simulink model "assembly_line"  (R2024b)
settings: Solver=VariableStepAuto  StartTime=0.0  StopTime=10.0  RelTol=1e-3
libraries: testLib x5
settings Model: Creator=AK123700  LastModifiedBy=AK123700

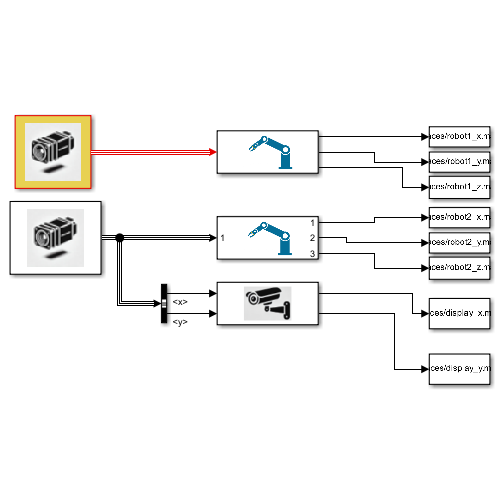
[thumbnail: Simulink's stored preview of the top-level diagram]
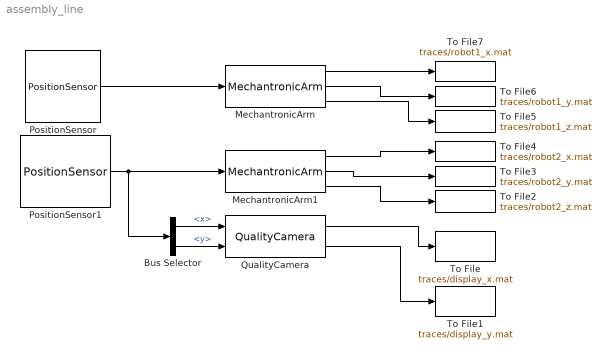
== system assembly_line ==
  Bus Selector : BusSelector  OutputSignals=x,y
  MechantronicArm : testLib/MechantronicArm  SystemSampleTime=-1  VariantActivationTime=update diagram  AllowFlexibleInterface=on  Latency=0  AutoFrameSizeCalculation=off
      mask Display: image('robot-icon.png', [0,0,0,0,80,80]);
  MechantronicArm1 : testLib/MechantronicArm  SystemSampleTime=-1  VariantActivationTime=update diagram  AllowFlexibleInterface=on  Latency=0  AutoFrameSizeCalculation=off
      mask Display: image('robot-icon.png', [0,0,0,0,80,80]);
  PositionSensor : testLib/PositionSensor  SystemSampleTime=-1  VariantActivationTime=update diagram  AllowFlexibleInterface=on  Latency=0  AutoFrameSizeCalculation=off
      mask Display: image('position-icon.png', [0,0,0,0,80,80]);
  PositionSensor1 : testLib/PositionSensor  SystemSampleTime=-1  VariantActivationTime=update diagram  AllowFlexibleInterface=on  Latency=0  AutoFrameSizeCalculation=off
      mask Display: image('position-icon.png', [0,0,0,0,80,80]);
  QualityCamera : testLib/QualityCamera  SystemSampleTime=-1  VariantActivationTime=update diagram  AllowFlexibleInterface=on  Latency=0  AutoFrameSizeCalculation=off
      mask Display: image('camera-icon.png', [0,0,0,0,80,80]);
  To File : ToFile  Filename=traces/display_x.mat  MatrixName=display_x_final  SaveFormat=Timeseries
  To File1 : ToFile  Filename=traces/display_y.mat  MatrixName=display_y_final  SaveFormat=Timeseries
  To File2 : ToFile  Filename=traces/robot2_z.mat  MatrixName=robot2_z_final  SaveFormat=Timeseries
  To File3 : ToFile  Filename=traces/robot2_y.mat  MatrixName=robot2_y_final  SaveFormat=Timeseries
  To File4 : ToFile  Filename=traces/robot2_x.mat  MatrixName=robot2_x_final  SaveFormat=Timeseries
  To File5 : ToFile  Filename=traces/robot1_z.mat  MatrixName=robot1_z_final  SaveFormat=Timeseries
  To File6 : ToFile  Filename=traces/robot1_y.mat  MatrixName=robot1_y_final  SaveFormat=Timeseries
  To File7 : ToFile  Filename=traces/robot1_x.mat  MatrixName=robot1_x_final  SaveFormat=Timeseries
  wires:
  QualityCamera/1 -> To File/1
  QualityCamera/2 -> To File1/1
  MechantronicArm1/3 -> To File2/1
  MechantronicArm1/1 -> To File4/1
  MechantronicArm1/2 -> To File3/1
  MechantronicArm/1 -> To File7/1
  MechantronicArm/2 -> To File6/1
  MechantronicArm/3 -> To File5/1
  PositionSensor/1 -> MechantronicArm/1
  PositionSensor1/1 -> MechantronicArm1/1, Bus Selector/1
  Bus Selector/1 -> QualityCamera/1  "<x>"
  Bus Selector/2 -> QualityCamera/2  "<y>"
